simulink model "nonlinear_closed_loop"  (R2023b)
settings: Solver=VariableStepAuto  StartTime=0.0  StopTime=20  MaxStep=0.01  RelTol=1e-5
undefined symbols (not defined in the file): K_act_b, K_act_f, u0, x0
libraries: simulink x2, cstblocks x2
settings Model: Creator=torb  LastModifiedBy=torb

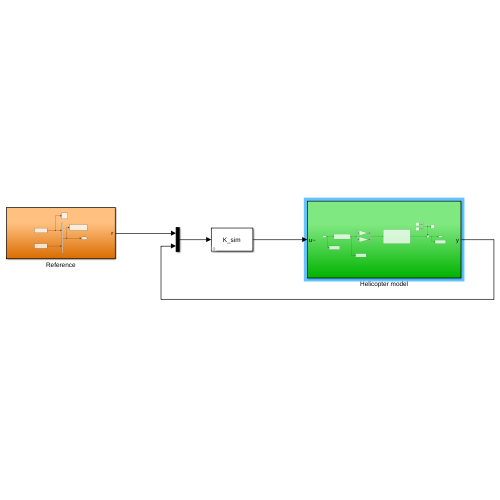
[thumbnail: Simulink's stored preview of the top-level diagram]
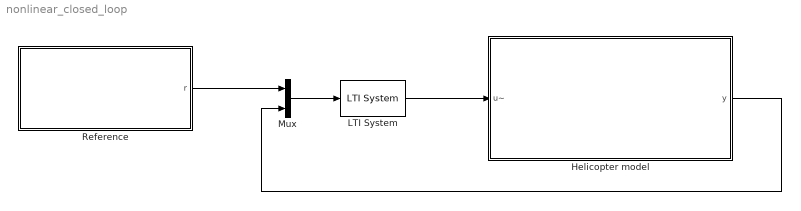
== system nonlinear_closed_loop ==
  Helicopter model : Subsystem
  LTI System : cstblocks/LTI System  sys=K_sim  IC=[]  PadeOrder=0
  Mux : Mux  Inputs=2
  Reference : Subsystem
  wires:
  Helicopter model/1(y) -> Mux/2
  Reference/1(r) -> Mux/1
  LTI System/1 -> Helicopter model/1(u~)
  Mux/1 -> LTI System/1

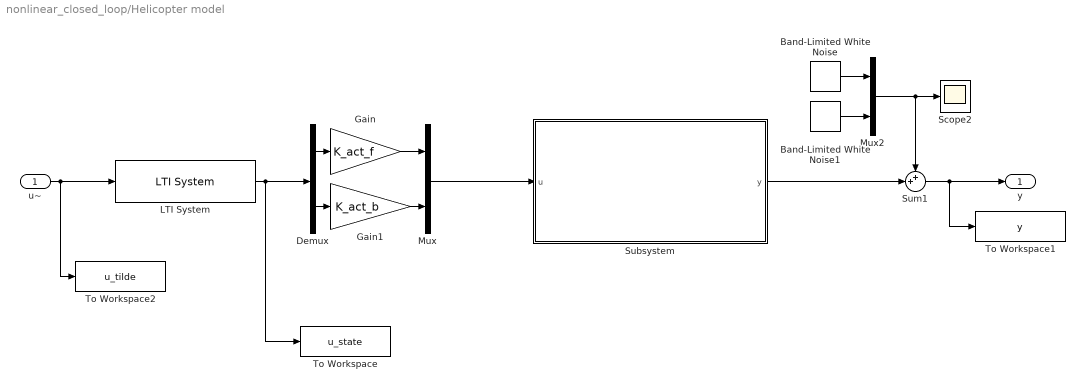
== system nonlinear_closed_loop/Helicopter model ==
  u~ : Inport
  Band-Limited White Noise : simulink/Sources/Band-Limited White Noise  Cov=noise_power  Ts=0.01  seed=[23341]
  Band-Limited White Noise1 : simulink/Sources/Band-Limited White Noise  Cov=noise_power  Ts=0.01  seed=[231]
  Demux : Demux  Outputs=2
  Gain : Gain  Gain=K_act_f
  Gain1 : Gain  Gain=K_act_b
  LTI System : cstblocks/LTI System  sys=G_act  IC=[]  PadeOrder=0
  Mux : Mux  Inputs=2
  Mux2 : Mux  Inputs=2
  Scope2 : Scope
  Subsystem : Subsystem
  Sum1 : Sum  Inputs=++|
  To Workspace : ToWorkspace  VariableName=u_state  SaveFormat=Timeseries  SampleTime=-1
  To Workspace1 : ToWorkspace  VariableName=y  SaveFormat=Timeseries  SampleTime=-1
  To Workspace2 : ToWorkspace  VariableName=u_tilde  SaveFormat=Timeseries  SampleTime=-1
  y : Outport
  wires:
  u~/1 -> To Workspace2/1, LTI System/1
  LTI System/1 -> Demux/1, To Workspace/1
  Demux/2 -> Gain1/1
  Demux/1 -> Gain/1
  Gain/1 -> Mux/1
  Gain1/1 -> Mux/2
  Band-Limited White Noise/1 -> Mux2/1
  Band-Limited White Noise1/1 -> Mux2/2
  Mux2/1 -> Sum1/1, Scope2/1
  Sum1/1 -> y/1, To Workspace1/1
  Mux/1 -> Subsystem/1(u)
  Subsystem/1(y) -> Sum1/2

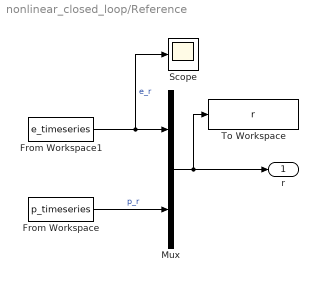
== system nonlinear_closed_loop/Reference ==
  From Workspace : FromWorkspace  VariableName=p_timeseries
  From Workspace1 : FromWorkspace  VariableName=e_timeseries
  Mux : Mux  Inputs=2
  Scope : Scope
  To Workspace : ToWorkspace  VariableName=r  SaveFormat=Timeseries  SampleTime=-1
  r : Outport
  wires:
  Mux/1 -> To Workspace/1, r/1
  From Workspace/1 -> Mux/2  "p_r"
  From Workspace1/1 -> Mux/1, Scope/1  "e_r"

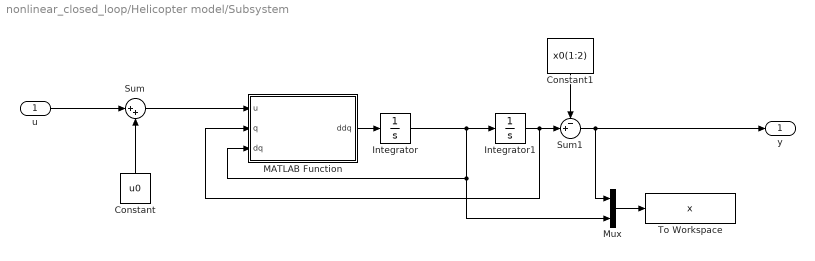
== system nonlinear_closed_loop/Helicopter model/Subsystem ==
  u : Inport
  Constant : Constant  Value=u0
  Constant1 : Constant  Value=x0(1:2)
  Integrator : Integrator
  Integrator1 : Integrator  InitialCondition=x0(1:2)
  MATLAB Function : MATLAB Function  TreatAsAtomicUnit=on
  Mux : Mux  Inputs=2
  Sum : Sum  Inputs=|++
  Sum1 : Sum  Inputs=-+|
  To Workspace : ToWorkspace  VariableName=x  SaveFormat=Timeseries  SampleTime=-1
  y : Outport
  wires:
  Mux/1 -> To Workspace/1
  Constant1/1 -> Sum1/1
  u/1 -> Sum/1
  Integrator/1 -> Mux/2, MATLAB Function/3(dq), Integrator1/1
  MATLAB Function/1(ddq) -> Integrator/1
  Constant/1 -> Sum/2
  Sum1/1 -> y/1, Mux/1
  Integrator1/1 -> Sum1/2, MATLAB Function/2(q)
  Sum/1 -> MATLAB Function/1(u)

== matlab function nonlinear_closed_loop/Helicopter model/Subsystem/MATLAB Function ==
  data: u input; ddq output size=2; q input; dq input
function ddq = rigid_body_dyn(u, q, dq)
    M = M_fun(q);
    b = b_fun(q, dq);
    g = g_fun(q);
    tau = tau_fun(q, u);

    lam = 0;
    ddq = (M + lam*eye(size(q, 1)))\(-b-g+tau);
end
